simulink model "P4_sim"  (R2020b)
settings: Solver=FixedStepAuto  StartTime=0.0  StopTime=25  FixedStep=0.01  RelTol=1e-3
model workspace (MAT data in the model file):
  eslasticidade = 0
  teste = 0
libraries: simulink x2
settings Model: Creator=Tiago  LastModifiedBy=Utilizador
settings SolverCC: ZeroCrossAlgorithm=Adaptive
settings DataIOCC: SaveState=on
settings DebuggingCC: IgnoredZcDiagnostic=none

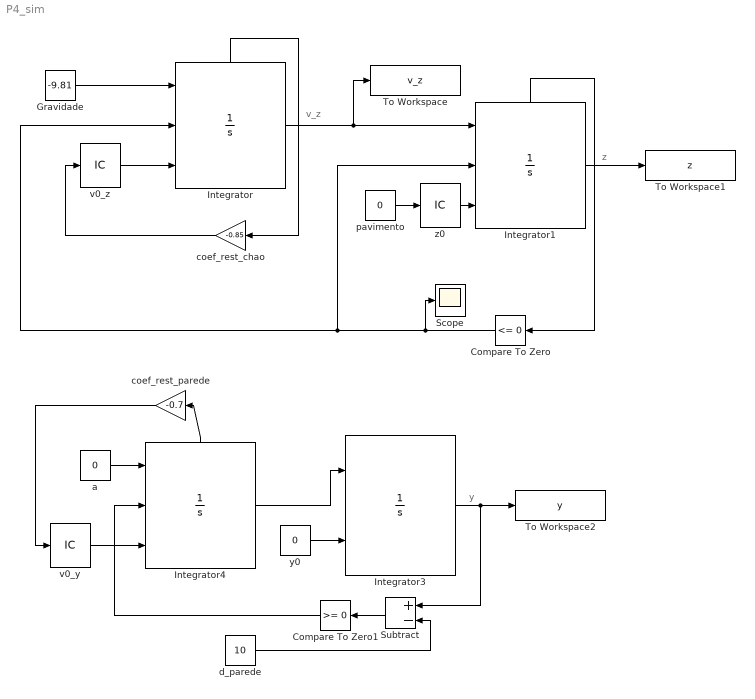
== system P4_sim ==
  note: z
  note: v_z
  note: y
  Compare To Zero : simulink/Logic and Bit Operations/Compare To Zero  relop=<=  OutDataTypeStr=boolean
  Compare To Zero1 : simulink/Logic and Bit Operations/Compare To Zero  relop=>=  OutDataTypeStr=boolean
  Gravidade : Constant  Value=-9.81
  Integrator : Integrator  ExternalReset=rising  InitialConditionSource=external  ShowStatePort=on  ContinuousStateAttributes='Velocidade'
  Integrator1 : Integrator  ExternalReset=rising  InitialConditionSource=external  ShowStatePort=on
  Integrator3 : Integrator  InitialConditionSource=external
  Integrator4 : Integrator  ExternalReset=rising  InitialConditionSource=external  ShowStatePort=on  ContinuousStateAttributes='Velocidade'
  Scope : Scope
  Subtract : Sum  Inputs=+-
  To Workspace : ToWorkspace  VariableName=v_z  SaveFormat=Timeseries  SampleTime=-1
  To Workspace1 : ToWorkspace  VariableName=z  SaveFormat=Timeseries  SampleTime=-1
  To Workspace2 : ToWorkspace  VariableName=y  SaveFormat=Timeseries  SampleTime=-1
  a : Constant  Value=0
  coef_rest_chao : Gain  Tag=teste  Gain=-0.85
  coef_rest_parede : Gain  Gain=-0.7
  d_parede : Constant  Value=10
  pavimento : Constant  Value=0
  v0_y : InitialCondition  Value=2
  v0_z : InitialCondition  Value=0
  y0 : Constant  Value=0
  z0 : InitialCondition  Value=10
  wires:
  Gravidade/1 -> Integrator/1
  v0_z/1 -> Integrator/3
  Integrator/State -> coef_rest_chao/1
  Integrator/1 -> To Workspace/1, Integrator1/1
  z0/1 -> Integrator1/3
  pavimento/1 -> z0/1
  Integrator1/State -> Compare To Zero/1
  Compare To Zero/1 -> Integrator/2, Integrator1/2, Scope/1
  Integrator1/1 -> To Workspace1/1
  Integrator3/1 -> Subtract/1, To Workspace2/1
  coef_rest_chao/1 -> v0_z/1
  Integrator4/1 -> Integrator3/1
  y0/1 -> Integrator3/2
  v0_y/1 -> Integrator4/3
  Integrator4/State -> coef_rest_parede/1
  coef_rest_parede/1 -> v0_y/1
  a/1 -> Integrator4/1
  d_parede/1 -> Subtract/2
  Subtract/1 -> Compare To Zero1/1
  Compare To Zero1/1 -> Integrator4/2
